simulink model "a2e1b"  (R2020a)
settings: Solver=VariableStepAuto  StartTime=0.0  StopTime=40.0  RelTol=1e-3
settings Model: Creator=mumun  LastModifiedBy=mumun
settings SolverCC: ZeroCrossAlgorithm=Adaptive
settings DebuggingCC: IgnoredZcDiagnostic=none

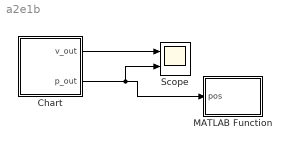
== system a2e1b ==
  Chart : Stateflow chart  TreatAsAtomicUnit=on
  MATLAB Function : MATLAB Function  TreatAsAtomicUnit=on
  Scope : Scope  NumInputPorts=2
  wires:
  Chart/2(p_out) -> MATLAB Function/1(pos), Scope/2
  Chart/1(v_out) -> Scope/1

== matlab function a2e1b/MATLAB Function ==
  data: pos input
function plottable(pos)

figure (1)
plot (pos(1,1), pos(1,2),'ro')
% hold on
% BorX=[0 0 2 2 0];
% BorY=[1 0 0 1 1];
% plot(BorX,BorY);
% hold on;
% area(BorX,BorY)
title('\bfBilliard Table','FontSize',14)
xlim([0 2])
ylim ([0 1])
grid on
box on

== stateflow chart a2e1b/Chart ==
  settings: updateMethod=CONTINUOUS  executeAtInitialization=1
  state Falling
    du:
    p_dot = v;
    v_dot = 0;
    p_out = p;
    v_out = v;
  (default) -> Falling : {initialize();}
  Falling -> Falling [order 1] : [boundarycrossing()]{resetposition()}
  Falling -> Falling [order 2] : [inhole()]
  data: yn function_output double; pocketed function_output double; v local double size=[1 2]; v_out output double size=[1 2]; p_out output double size=[1 2]; tableLen local double; tableWid local double; p local double size=[1 2]; holesize local double
  data v settings: updateMethod=SF_CONTINUOUS_TIME_DATA
  data p settings: updateMethod=SF_CONTINUOUS_TIME_DATA
  function initialize:
    | function initialize
    | 
    | p = [1 2]; %initial position of the ball in the board 
    | v = [1 1]; %initial velocity of the ball in x-y direction
    | tableLen= 2; %length of the table
    | tableWid= 1; %width of the table
    | holesize = 0.05; %d= 5 cm
    | 
    | end
  function resetposition:
    | function resetposition
    | 
    | if p(1,1) < 0
    |     p(1,1) = -p(1,1);
    |     v(1,1) = -1*v(1,1);
    |     v(1,2) = 1*v(1,2);
    | elseif p(1,1) > tableLen
    |     p(1,1) = 2*tableLen-p(1,1);
    |     v(1,1) = -1*v(1,1);
    |     v(1,2) = 1*v(1,2);
    | end
    | if p(1,2) < 0
    |     p(1,2) = -p(1,2);
    |     v(1,2) = -1*v(1,2);
    |     v(1,1) = 1*v(1,1);
    | elseif p(1,2) > tableWid
    |     p(1,2) = 2*tableWid-p(1,2);
    |     v(1,2) = -1*v(1,2);
    |     v(1,1) = 1*v(1,1);
    |    
    | end
  function yn = boundarycrossing:
    | function yn = boundarycrossing
    | 
    | if  p(1,1) < 0 || p(1,1) > tableLen || ...
    |     p(1,2) < 0 || p(1,2) > tableWid
    |     
    |     yn = 1;
    |     return;
    | end      
    | yn = 0;
  function pocketed = inhole:
    | function pocketed = inhole
    | 
    | if norm (p-[0 0]) < holesize
    |     pocketed = 1;
    | elseif norm (p-[tableLen 0]) < holesize
    |     pocketed = 1;
    | elseif norm (p-[0 tableWid]) < holesize
    |     pocketed = 1;
    | elseif norm (p-[tableLen tableWid]) < holesize
    |     pocketed = 1;
    | else
    |     pocketed = 0;
    |     
    | end
    | end
